simulink model "HybridModel_Phasor"  (R2018b)
settings: Solver=ode45  StartTime=0.0  StopTime=30  RelTol=1e-3
undefined symbols (not defined in the file or in its folder): A, B, C, D1, D11, Dd, Delta, j, to, V2G
libraries: powerlib x32, powerlib_meascontrol x28, simulink x2, re_lib x1
(part 1 of 4)
settings Model: Creator=Eduardo  LastModifiedBy=Eduardo

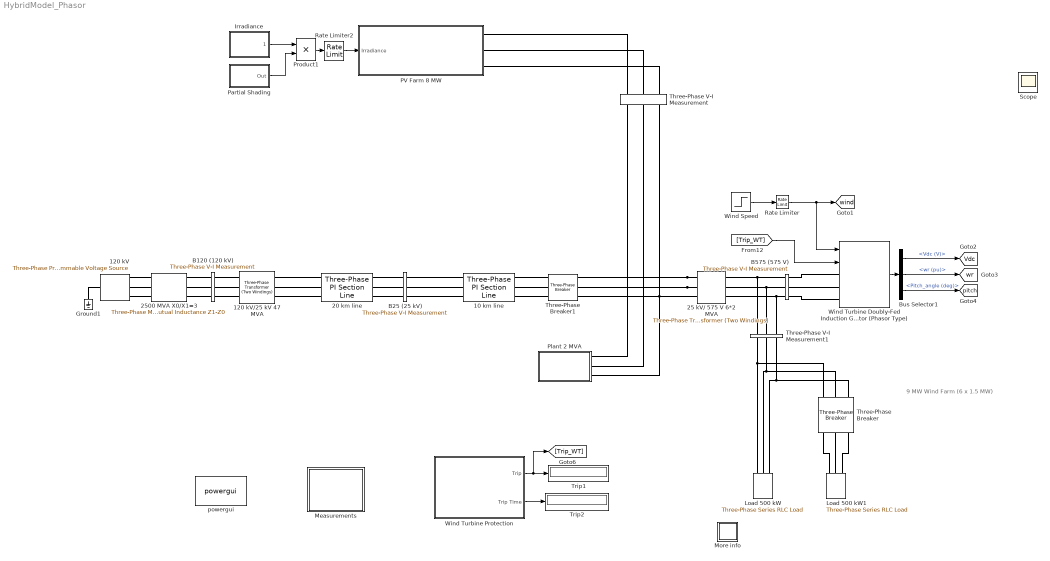
== system HybridModel_Phasor ==
  note: 9 MW Wind Farm
      | (6 x 1.5 MW)
  10 km line : powerlib/Elements/Three-Phase PI Section Line  LConnTagsString=a|b|c  RConnTagsString=A|B|C  Frequency=60  Resistances=[0.1153 0.413]  Inductances=[1.05e-3 3.32e-3]  Capacitances=[11.33e-009 5.01e-009]  Length=10
      settings: SourceProductName=Simscape Electrical
  120 kV : powerlib/Electrical Sources/Three-Phase Programmable Voltage Source  PositiveSequence=[120e3 0 60]  VariationEntity=None  VariationType=Step  VariationTypeAlt=Step  VariationStep=-0.15  VariationRate=10  VariationMagnitude=0.3  VariationFrequency=2  VariationTiming=[5 5.5]  VariationPhaseA=off  Amplitudes=[1 0.8 1.2 1.0]  TimeValues=[0 0.1 0.15 0.2]  HarmonicGeneration=off  HarmonicA=[1 -0.1 0 1]  HarmonicB=[2 0.15 35 2]  Timing="[5  5.5]"  BusType=swing  Pref=1e3  Qref=0  Qmin=-inf  Qmax=inf
      settings: SourceProductName=Simscape Electrical
  120 kV/25 kV 47 MVA : powerlib/Elements/Three-Phase Transformer (Two Windings)  Winding1Connection=Yg  Winding2Connection=Delta (D1)  CoreType=Three single-phase transformers  SetSaturation=off  Hysteresis=off  DataFile='basic_model'  SetInitialFlux=off  Measurements=None  UNITS=pu  NominalPower=[47e6 60 ]  Winding1="[ 120e3  0.08/30   0.08 ]"  Winding2="[ 25e3  0.08/30  0.08]"  Rm=500  Lm=500  L0=0.5  Saturation="[ 0,0  ;  0.005,1.2  ;  1.0,1.4 ]"  InitialFluxes=[ 0.8 , -0.8 , 0.7 ]  MoreParameters=off  BreakLoop=off  DataType=off  TransfoNumber=0
      settings: SourceProductName=Simscape Electrical
  20 km line : powerlib/Elements/Three-Phase PI Section Line  LConnTagsString=a|b|c  RConnTagsString=A|B|C  Frequency=60  Resistances=[0.1153 0.413]  Inductances=[1.05e-3 3.32e-3]  Capacitances=[11.33e-009 5.01e-009]  Length=20
      settings: SourceProductName=Simscape Electrical
  25 kV/ 575 V 6*2 MVA : powerlib/Elements/Three-Phase Transformer (Two Windings)  Winding1Connection=Yg  Winding2Connection=Delta (D1)  CoreType=Three single-phase transformers  SetSaturation=off  Hysteresis=off  DataFile='hysteresis'  SetInitialFlux=off  Measurements=None  UNITS=pu  NominalPower="[2e6*6  60]"  Winding1=[25e3 , 0.025/30 , 0.025]  Winding2=[ 575, 0.025/30 , 0.025]  Rm=500  Lm=inf  L0=0.5  Saturation=[ 0,0 ; 0.0024,1.2 ; 1.0,1.52 ]  InitialFluxes=[ 0.8 , -0.8 , 0.7 ]  MoreParameters=off  BreakLoop=off  DataType=off  TransfoNumber=0
      settings: SourceProductName=Simscape Electrical
  2500 MVA X0/X1=3 : powerlib/Elements/Three-Phase Mutual Inductance Z1-Z0  LConnTagsString=a|b|c  RConnTagsString=A|B|C  PositiveSequence="[0.1  1.0/(2*pi*60)] *120e3^2/2500e6"  ZeroSequence="[0.3  3.0/(2*pi*60)] *120e3^2/2500e6"
      settings: SourceProductName=Simscape Electrical  SourceProductBaseCode=PS
  B120 (120 kV) : powerlib/Measurements/Three-Phase V-I Measurement  VoltageMeasurement=phase-to-ground  SetLabelV=on  LabelV=Vabc_B120  Vpu=on  VpuLL=off  CurrentMeasurement=no  SetLabelI=on  LabelI=Iabc_B120  Ipu=off  Pbase=100e6  Vbase=120e3  OutputType=Complex  PhasorSimulation=on  PSBequivalent=0
      settings: SourceProductName=Simscape Electrical
  B25 (25 kV) : powerlib/Measurements/Three-Phase V-I Measurement  VoltageMeasurement=phase-to-ground  SetLabelV=on  LabelV=Vabc_B25  Vpu=on  VpuLL=off  CurrentMeasurement=yes  SetLabelI=on  LabelI=Iabc_B25  Ipu=on  Pbase=10e6  Vbase=25e3  OutputType=Complex  PhasorSimulation=on  PSBequivalent=0
      settings: SourceProductName=Simscape Electrical
  B575 (575 V) : powerlib/Measurements/Three-Phase V-I Measurement  VoltageMeasurement=phase-to-ground  SetLabelV=on  LabelV=Vabc_B575  Vpu=on  VpuLL=off  CurrentMeasurement=yes  SetLabelI=on  LabelI=Iabc_B575  Ipu=on  Pbase=6*1.5e6/0.9  Vbase=575  OutputType=Complex  PhasorSimulation=on  PSBequivalent=0
      settings: SourceProductName=Simscape Electrical
  Bus Selector1 : BusSelector  OutputSignals=Vdc (V),wr (pu),Pitch_angle (deg)
  Ground1 : powerlib/Elements/Ground  LConnTagsString=a
      settings: SourceProductName=Simscape Electrical
  Irradiance : Subsystem
      mask init:
      | load power_V2G
      mask Display: plot(V2G.IRRADIANCE.time,V2G.IRRADIANCE.SUN)
  Load 500 kW : powerlib/Elements/Three-Phase Series RLC Load  LConnTagsString=A|B|C  Configuration=Y (grounded)  NominalVoltage=575  Vabc=[1e3 1e3 1e3]  Vabcp=[1e3 1e3 1e3]  NominalFrequency=60  UnbalancedPower=off  ActivePower=500e3  InductivePower=0  CapacitivePower=0  Pabc=[10e3 9e3 11e3]  QLabc=[100 90 110]  QCabc=[100 90 110]  Pabcp=[10e3 9e3 11e3]  QLabcp=[100 90 110]  QCabcp=[100 90 110]  Measurements=None  LoadType=constant Z
      settings: SourceProductName=Simscape Electrical
  Load 500 kW1 : powerlib/Elements/Three-Phase Series RLC Load  LConnTagsString=A|B|C  Configuration=Y (grounded)  NominalVoltage=575  Vabc=[1e3 1e3 1e3]  Vabcp=[1e3 1e3 1e3]  NominalFrequency=60  UnbalancedPower=off  ActivePower=2e6  InductivePower=0  CapacitivePower=0  Pabc=[10e3 9e3 11e3]  QLabc=[100 90 110]  QCabc=[100 90 110]  Pabcp=[10e3 9e3 11e3]  QLabcp=[100 90 110]  QCabcp=[100 90 110]  Measurements=None  LoadType=constant Z
      settings: SourceProductName=Simscape Electrical
  Measurements : Subsystem
  More info : Subsystem
      settings: OpenFcn=showdemo(bdroot(gcb))
      mask Display: disp('?')
  PV Farm 8 MW : Subsystem  mask{eff=10, area=8e4}
      mask prompts: eff "Efficiency (%)"; area "Area (m^2)"
      mask help: The product of the effeciency, the area covered by the Pv farm and the irradiance in w/m2 will give you the power generate by the PV farm.
      mask DialogControl DescGroupVar Prompt: PV farm
      mask DialogControl DescTextVar Prompt: The product of the efficiency, the area covered by the PV farm and the irradiance in W/m2 will give you the power generated by the PV farm.
      mask Display: image(imread('panel.jpg'))
  Partial Shading : Subsystem  mask(Signal Disturbance){Hour=12, Minute=0, Second=0, Duration=5*60, Factor=0.7}
      mask prompts: Duration "Duration (s):"
      mask help: Within the specified time range defined by Start and Duration parameters, output is set to 'Factor'. Outside the specified time range output is kept at 1.0.
      mask init:
      | T2=(Hour-1)*60*60;    % Hour in seconds
      | T3=(Minute-1)*60;  % Minute in seconds
      | Ton=T2+T3+(Second-1);    % Beginning of fault (s)
      | Toff=Ton+Duration; % End of fault (s)
      mask TypeOptions Hour: 0 |      1 |      2 |      3 |      4 |      5 |      6 |      7 |      8 |      9 |     10 |     11 |     12 |     13 |     14 |     15 |     16 |     17 |     18 |     19 |     20 |     21 |     22 |     23
      mask TypeOptions Minute: 0 |      1 |      2 |      3 |      4 |      5 |      6 |      7 |      8 |      9 |     10 |     11 |     12 |     13 |     14 |     15 |     16 |     17 |     18 |     19 |     20 |     21 |     22 |     23 |     24 |     25 |     26 |     27 |     28 |     29 |     30 |     31 |     32 |     33 |     34 |     35 |     36 |     37 |     38 |     39 |     40 |     41 |     42 |     43 |     44 |     45 |     46 |     47 |     48 |     49 |     50 |     51 |     52 |     53 |     54 |     55 |     56 |     57 |     58 |     59
      mask TypeOptions Second: 0 |      1 |      2 |      3 |      4 |      5 |      6 |      7 |      8 |      9 |     10 |     11 |     12 |     13 |     14 |     15 |     16 |     17 |     18 |     19 |     20 |     21 |     22 |     23 |     24 |     25 |     26 |     27 |     28 |     29 |     30 |     31 |     32 |     33 |     34 |     35 |     36 |     37 |     38 |     39 |     40 |     41 |     42 |     43 |     44 |     45 |     46 |     47 |     48 |     49 |     50 |     51 |     52 |     53 |     54 |     55 |     56 |     57 |     58 |     59
      mask DialogControl Control2 Prompt: Start:
  Plant 2 MVA : Subsystem
  Product1 : Product
  Rate Limiter : RateLimiter
  Rate Limiter2 : RateLimiter  RisingSlewLimit=1e4  FallingSlewLimit=-1e4  SampleTimeMode=inherited
  Scope : Scope  NumInputPorts=3
  Three-Phase V-I Measurement : powerlib/Measurements/Three-Phase V-I Measurement  VoltageMeasurement=phase-to-ground  SetLabelV=on  LabelV=V_PV  Vpu=off  VpuLL=off  CurrentMeasurement=yes  SetLabelI=on  LabelI=I_PV  Ipu=off  Pbase=100e6  Vbase=500e3  OutputType=Complex  PhasorSimulation=on  PSBequivalent=0
  Three-Phase V-I Measurement1 : powerlib/Measurements/Three-Phase V-I Measurement  VoltageMeasurement=phase-to-ground  SetLabelV=on  LabelV=Vabc_load  Vpu=off  VpuLL=off  CurrentMeasurement=yes  SetLabelI=on  LabelI=Iabc_load  Ipu=off  Pbase=100e6  Vbase=500e3  OutputType=Complex  PhasorSimulation=on  PSBequivalent=0
  Three-Phase Breaker : powerlib/Elements/Three-Phase Breaker  InitialState=open  SwitchA=on  SwitchB=on  SwitchC=on  SwitchTimes=[5 15]  External=off  BreakerResistance=0.01  SnubberResistance=1e6  SnubberCapacitance=inf  Measurements=None
  Three-Phase Breaker1 : powerlib/Elements/Three-Phase Breaker  InitialState=closed  SwitchA=on  SwitchB=on  SwitchC=on  SwitchTimes="[20  60]"  External=off  BreakerResistance=0.01  SnubberResistance=1e6  SnubberCapacitance=inf  Measurements=None
  Trip1 : Display
  Trip2 : Display
  Wind Speed : Step  Time=5  Before=8  After=8  SampleTime=0
  Wind Turbine Doubly-Fed Induction Generator (Phasor Type) : re_lib/Wind Generation/Wind Turbine Doubly-Fed Induction Generator (Phasor Type)  ExternalTm=off  nom=[6*1.5e6/0.9 575 60]  sta=[ 0.00706 0.171]  rot=[ 0.005 0.156]  Lm=2.9  mec=[5.04 0.01 3]  init=[0.2 0 0 0 0 0]  speed_power=[0 0; 0.24 0.007; 0.36 0.024; 0.6 0.112; 0.96 0.46; 1.2 0.898; 1.5 0.898]  Pmec=6*1.5e6  speed_ABCD=[0.7 0.71 1.2 1.21]  power_C=0.73  wind_point_C=12  pitch_gain=500  pitch_max=45  pitch_rate=2  Pmax=0.5  Lchoke=[0.15 0.15/100]  init_inductor=[0 90]  Vdc_nom=1200  capacitor=6*10000e-6  ControlVQ=Voltage regulation  Vref=1.0  ExternalVref=off  Qref=0  ExternalQref=off  Iq_ref=0  ExternalIqref=off  Kpi_volt_reg=[1.25 300]  Xs=0.02  Kpi_Q=[0.05 5]  Kpi_power_reg=[1 100]  Kpi_dc_reg=[0.002 0.05]  Kpi_grid_side_cur_reg=[1 100]  Kpi_rotor_side_cur_reg=[0.3 8]  V_slew_rate=100  Q_slew_rate=100  power_slew_rate=1  current_slew_rate=200
      settings: SourceProductName=Simscape Electrical  SourceProductBaseCode=PS
  Wind Turbine Protection : Subsystem
      mask Display: disp('Wind\nTurbine\nProtection')
  powergui : powerlib/powergui  Priority=2  SimulationMode=Phasor  SampleTime=5e-6  frequency=60  Iterations=50  frequencyindice=60  Pbase=100e6  ErrMax=1e-4  UnitsV=kV  UnitsW=MW  buscounter=0  FunctionMessages=off  echomessages=off  EnableUseOfTLC=off  CurrentSourceSwitches=off  DisableSnubberDevices=off  DisableRonSwitches=off  DisableVfSwitches=off  DisplayEquations=off  SolverType=Tustin/Backward Euler (TBE)  Interpol=off  ExternalGateDelay=off  methode=off  Ts=100  x0status=blocks  SPID=off  SwTol=0  HookPort=off  RestoreLinks=warning  ResistiveCurrentMeasurement=off  Frange=[0:2:500]  Ylog=off  Xlog=off  ShowGrid=off  save=off  variable=ZData  structure=0  ZoomFFT=on  StartTime=0.0  cycles=1  DisplayStyle=1  fundamental=60  FreqAxis=off  MaxFrequency=1000  frequencyindicesteady=1  RmsSteady=1  display=off
  tag scope: Vdc=global, pitch=global, wind=global, wr=global
  wires:
  Wind Speed/1 -> Rate Limiter/1
  Rate Limiter/1 -> Wind Turbine Doubly-Fed Induction Generator (Phasor Type)/1, [wind]
  Wind Turbine Protection/2(Trip Time) -> Trip2/1
  Wind Turbine Protection/1(Trip) -> [Trip_WT], Trip1/1
  Wind Turbine Doubly-Fed Induction Generator (Phasor Type)/1 -> Bus Selector1/1
  Bus Selector1/2 -> [wr]  "<wr (pu)>"
  Bus Selector1/1 -> [Vdc]  "<Vdc (V)>"
  Bus Selector1/3 -> [pitch]  "<Pitch_angle (deg)>"
  [Trip_WT] -> Wind Turbine Doubly-Fed Induction Generator (Phasor Type)/2
  ? -> ?
  Product1/1 -> Rate Limiter2/1
  Rate Limiter2/1 -> PV Farm 8 MW/1(Irradiance)
  Partial Shading/1(Out) -> Product1/2
  Irradiance/1(" ") -> Product1/1
  connections:
  B25 (25 kV)/RConn1 -- 10 km line/LConn1
  B25 (25 kV)/RConn2 -- 10 km line/LConn2
  B25 (25 kV)/RConn3 -- 10 km line/LConn3
  B575 (575 V)/LConn2 -- Three-Phase V-I Measurement1/RConn2 -- 25 kV/ 575 V 6*2 MVA/RConn2
  B575 (575 V)/LConn1 -- Three-Phase V-I Measurement1/RConn1 -- 25 kV/ 575 V 6*2 MVA/RConn1
  120 kV/25 kV 47 MVA/RConn2 -- 20 km line/LConn2
  120 kV/25 kV 47 MVA/RConn3 -- 20 km line/LConn3
  Load 500 kW/LConn3 -- Three-Phase V-I Measurement1/LConn3 -- Three-Phase Breaker/RConn3
  120 kV/25 kV 47 MVA/RConn1 -- 20 km line/LConn1
  B25 (25 kV)/LConn1 -- 20 km line/RConn1
  B575 (575 V)/RConn2 -- Wind Turbine Doubly-Fed Induction Generator (Phasor Type)/LConn2
  120 kV/RConn1 -- 2500 MVA X0/X1=3/LConn1
  B120 (120 kV)/RConn2 -- 120 kV/25 kV 47 MVA/LConn2
  B120 (120 kV)/LConn2 -- 2500 MVA X0/X1=3/RConn2
  B120 (120 kV)/LConn3 -- 2500 MVA X0/X1=3/RConn3
  B120 (120 kV)/RConn1 -- 120 kV/25 kV 47 MVA/LConn1
  20 km line/RConn3 -- B25 (25 kV)/LConn3
  B575 (575 V)/RConn1 -- Wind Turbine Doubly-Fed Induction Generator (Phasor Type)/LConn1
  120 kV/RConn3 -- 2500 MVA X0/X1=3/LConn3
  B575 (575 V)/RConn3 -- Wind Turbine Doubly-Fed Induction Generator (Phasor Type)/LConn3
  120 kV/RConn2 -- 2500 MVA X0/X1=3/LConn2
  20 km line/RConn2 -- B25 (25 kV)/LConn2
  Ground1/LConn1 -- 120 kV/LConn1
  B120 (120 kV)/LConn1 -- 2500 MVA X0/X1=3/RConn1
  B120 (120 kV)/RConn3 -- 120 kV/25 kV 47 MVA/LConn3
  Plant 2 MVA/LConn3 -- 25 kV/ 575 V 6*2 MVA/LConn3 -- Three-Phase Breaker1/RConn3 -- Three-Phase V-I Measurement/RConn3
  25 kV/ 575 V 6*2 MVA/LConn1 -- Plant 2 MVA/LConn1 -- Three-Phase Breaker1/RConn1 -- Three-Phase V-I Measurement/RConn1
  25 kV/ 575 V 6*2 MVA/LConn2 -- Plant 2 MVA/LConn2 -- Three-Phase Breaker1/RConn2 -- Three-Phase V-I Measurement/RConn2
  Load 500 kW1/LConn1 -- Three-Phase Breaker/LConn1
  Load 500 kW1/LConn2 -- Three-Phase Breaker/LConn2
  Load 500 kW1/LConn3 -- Three-Phase Breaker/LConn3
  PV Farm 8 MW/RConn1 -- Three-Phase V-I Measurement/LConn1
  PV Farm 8 MW/RConn2 -- Three-Phase V-I Measurement/LConn2
  PV Farm 8 MW/RConn3 -- Three-Phase V-I Measurement/LConn3
  Three-Phase Breaker1/LConn1 -- 10 km line/RConn1
  Three-Phase Breaker1/LConn3 -- 10 km line/RConn3
  Three-Phase Breaker1/LConn2 -- 10 km line/RConn2
  Load 500 kW/LConn1 -- Three-Phase V-I Measurement1/LConn1 -- Three-Phase Breaker/RConn1
  Load 500 kW/LConn2 -- Three-Phase V-I Measurement1/LConn2 -- Three-Phase Breaker/RConn2
  B575 (575 V)/LConn3 -- Three-Phase V-I Measurement1/RConn3 -- 25 kV/ 575 V 6*2 MVA/RConn3

== system HybridModel_Phasor/Irradiance ==
  1-D Lookup IRRADIANCE Table : Lookup_n-D  NumberOfTableDimensions=1  BreakpointsForDimension1=V2G.IRRADIANCE.time  BeginIndexSearchUsingPreviousIndexResult=on  Table=V2G.IRRADIANCE.SUN  InternalRulePriority=Speed  RndMeth=Simplest  InputSameDT=on
  Add : Sum
  Clock1 : Clock
  Constant1 : Constant
  Second-->Hour : Gain  Gain=1/(60*60)
  " " : Outport
  wires:
  Constant1/1 -> Add/2
  Add/1 -> 1-D Lookup IRRADIANCE Table/1  "Hour of the day"
  1-D Lookup IRRADIANCE Table/1 -> " "/1
  Clock1/1 -> Second-->Hour/1
  Second-->Hour/1 -> Add/1

== system HybridModel_Phasor/Measurements ==
  Grid : Scope  NumInputPorts=8
  Grid Data acquisition : Subsystem
  PV : Scope  NumInputPorts=4
  PV Array DATA : Subsystem
  Wind Turbine : Scope  NumInputPorts=8
  Wind turbine Data acquisition : Subsystem
  wires:
  Wind turbine Data acquisition/3(P_mean) -> Wind Turbine/3  "Generated P(MW)"
  Grid Data acquisition/1("Vabc_B120 ") -> Grid/1  "Vabc_B120 (pu)"
  Grid Data acquisition/2("Vabc_B25 ") -> Grid/2  "Vabc_B25 (pu)"
  Grid Data acquisition/3("Vabc_B575 ") -> Grid/3  "Vabc_B575 (pu)"
  Grid Data acquisition/4(P_B25) -> Grid/4  "P_B25 (MW)"
  Grid Data acquisition/5(Q_B25) -> Grid/5  "Q_B25 (Mvar)"
  [Vdc] -> Wind Turbine/5  "Vdc (V)"
  [wr] -> Wind Turbine/6  "Speed (pu)"
  Wind turbine Data acquisition/1(V1_B575) -> Wind Turbine/1  "Pos. seq. V1_B575 (pu)"
  Wind turbine Data acquisition/2(I1_B575) -> Wind Turbine/2  "Pos. seq. I1_B575 (pu)"
  Wind turbine Data acquisition/4(Q_mean) -> Wind Turbine/4  "Generated Q(Mvar)"
  Grid Data acquisition/8(Motor_Speed) -> Grid/8  "Motor Speed (pu)"
  Grid Data acquisition/7(I1_Plant) -> Grid/7  "I Plant pos. seq. (pu/2 MVA)"
  Grid Data acquisition/6(V1_Plant) -> Grid/6  "V_Plant 2.3kV pos. seq. (pu)"
  [wind] -> Wind Turbine/7  "Wind speed (m/s)"
  [pitch] -> Wind Turbine/8  "pitch angle (deg)"
  PV Array DATA/2(I_PV) -> PV/2  "Pos. seq. I1_B575 (pu)"
  PV Array DATA/3(P_mean) -> PV/3  "Generated P(MW)"
  PV Array DATA/4(Q_mean) -> PV/4  "Generated Q(Mvar)"
  PV Array DATA/1(V_PV) -> PV/1  "Pos. seq. V1_B575 (pu)"

== system HybridModel_Phasor/More info ==

== system HybridModel_Phasor/PV Farm 8 MW ==
  Irradiance : Inport
  PV Farm : Subsystem
  PV farm : Scope  NumInputPorts=2
  "Power (3ph, Phasor)2" : powerlib_meascontrol/Measurements/Power (3ph, Phasor)
      settings: SourceProductName=Simscape Power Systems  SourceProductBaseCode=PS
  VabcPV : powerlib/Measurements/Three-Phase V-I Measurement  VoltageMeasurement=phase-to-ground  SetLabelV=on  LabelV=V_Solar  Vpu=off  VpuLL=off  CurrentMeasurement=yes  SetLabelI=on  LabelI=I_Solar  Ipu=off  Pbase=2*1.5e6/0.9  Vbase=25e3  OutputType=Complex  PhasorSimulation=on  PSBequivalent=0
  A : PMIOPort  Side=Right
  B : PMIOPort  Port=2  Side=Right
  C : PMIOPort  Port=3  Side=Right
  tag scope: Solar_Power=global
  wires:
  Irradiance/1 -> PV Farm/1(irradiance)
  [V_Solar] -> "Power (3ph, Phasor)2"/1
  "Power (3ph, Phasor)2"/1 -> [Solar_Power], PV farm/1  "P(W)"
  [I_Solar] -> "Power (3ph, Phasor)2"/2
  "Power (3ph, Phasor)2"/2 -> PV farm/2  "Q(VA)"
  connections:
  B/RConn1 -- VabcPV/RConn2
  VabcPV/LConn2 -- PV Farm/RConn2
  A/RConn1 -- VabcPV/RConn1
  VabcPV/RConn3 -- C/RConn1
  PV Farm/RConn1 -- VabcPV/LConn1
  VabcPV/LConn3 -- PV Farm/RConn3

== system HybridModel_Phasor/Partial Shading ==
  Add : Sum
  Clock : Clock
  Compare To Constant : simulink/Logic and Bit Operations/Compare To Constant  relop=>=  const=Ton  OutDataTypeStr=boolean
  Compare To Constant1 : simulink/Logic and Bit Operations/Compare To Constant  relop=<  const=Toff  OutDataTypeStr=boolean
  Constant : Constant  Value=Factor
  Logical Operator : Logic  AllPortsSameDT=off  OutDataTypeStr=float('double')
  Logical Operator1 : Logic  Operator=NOT  AllPortsSameDT=off  OutDataTypeStr=float('double')
  Product : Product
  Out : Outport
  wires:
  Add/1 -> Out/1
  Product/1 -> Add/2
  Constant/1 -> Product/2
  Compare To Constant/1 -> Logical Operator/1
  Clock/1 -> Compare To Constant1/1, Compare To Constant/1
  Compare To Constant1/1 -> Logical Operator/2
  Logical Operator/1 -> Logical Operator1/1, Product/1
  Logical Operator1/1 -> Add/1

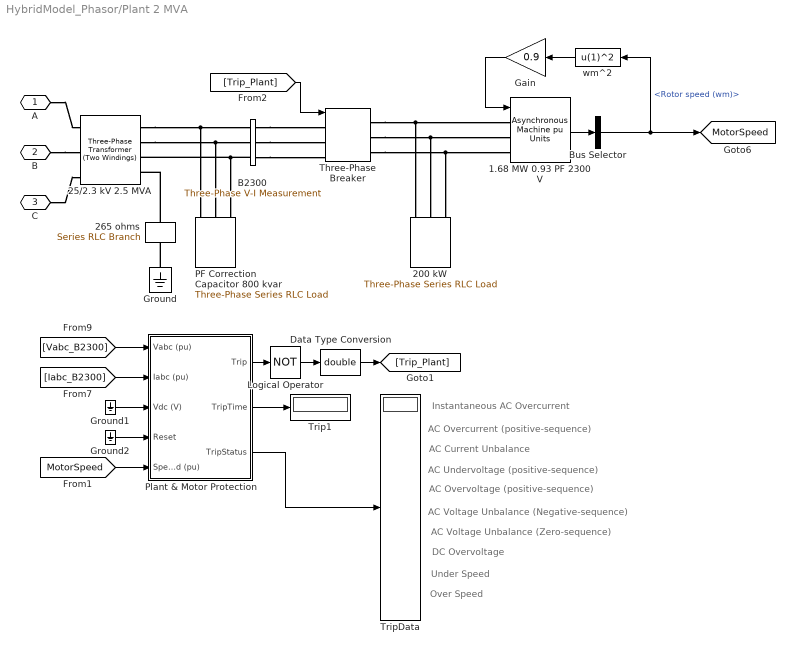
== system HybridModel_Phasor/Plant 2 MVA ==
  note: Instantaneous AC Overcurrent
  note: AC Overcurrent (positive-sequence)
  note: AC Current Unbalance
  note: AC Undervoltage (positive-sequence)
  note: AC Overvoltage (positive-sequence)
  note: AC Voltage Unbalance (Negative-sequence)
  note: AC Voltage Unbalance (Zero-sequence)
  note: DC Overvoltage
  note: Under Speed
  note: Over Speed
  1.68 MW 0.93 PF 2300 V : powerlib/Machines/Asynchronous Machine pu Units  RotorType=Squirrel-cage  PresetModel=No  MechanicalLoad=Torque Tm  ShowDetailedParameters=on  ReferenceFrame=Rotor  Units=pu  MeasurementBus=off  NominalParameters=[1.68e6/0.93 2300 60]  Stator=[0.0092 0.0717]  Rotor=[0.007 0.0717]  Cage1=[0.01909 0.0397]  Cage2=[0.01909 0.0397]  Lm=4.14  Mechanical=[0.5 0 2]  PolePairs=2  InitialConditions="[ 1e-3,0   0,0,0   0,0,0 ]"  SimulateSaturation=off  Saturation=[ 0 0 ; 0 0 ]  LoadFlowParameters=0  TsPowergui=0  TsBlock=-1  IterativeModel=Forward Euler  IterativeDiscreteModel=Trapezoidal non iterative  Pmec=3e3
      settings: SourceProductName=Simscape Electrical  SourceProductBaseCode=PS
  200 kW : powerlib/Elements/Three-Phase Series RLC Load  LConnTagsString=A|B|C  Configuration=Y (grounded)  NominalVoltage=2300  Vabc=[1e3 1e3 1e3]  Vabcp=[1e3 1e3 1e3]  NominalFrequency=60  UnbalancedPower=off  ActivePower=200e3  InductivePower=0  CapacitivePower=0  Pabc=[10e3 9e3 11e3]  QLabc=[100 90 110]  QCabc=[100 90 110]  Pabcp=[10e3 9e3 11e3]  QLabcp=[100 90 110]  QCabcp=[100 90 110]  Measurements=None  LoadType=constant Z
      settings: SourceProductName=Simscape Electrical
  25/2.3 kV 2.5 MVA : powerlib/Elements/Three-Phase Transformer (Two Windings)  Winding1Connection=Delta (D11)  Winding2Connection=Yn  CoreType=Three single-phase transformers  SetSaturation=off  Hysteresis=off  DataFile='basic_model'  SetInitialFlux=off  Measurements=None  UNITS=pu  NominalPower=[2.5e6 60 ]  Winding1="[ 25e3  0.04/30   0.04 ]"  Winding2="[ 2.3e3  0.04/30  0.04]"  Rm=500  Lm=500  L0=0.5  Saturation="[ 0,0  ;  0.005,1.2  ;  1.0,1.4 ]"  InitialFluxes=[ 0.8 , -0.8 , 0.7 ]  MoreParameters=off  BreakLoop=off  DataType=off  TransfoNumber=0
      settings: SourceProductName=Simscape Electrical
  265 ohms : powerlib/Elements/Series RLC Branch  LConnTagsString=__new0  RConnTagsString=__new0  BranchType=R  Resistance=265  Inductance=1.0  SetiL0=off  InitialCurrent=0  Capacitance=1.0  Setx0=off  InitialVoltage=0  Measurements=None
      settings: SourceProductName=Simscape Electrical
  B2300 : powerlib/Measurements/Three-Phase V-I Measurement  VoltageMeasurement=phase-to-ground  SetLabelV=on  LabelV=Vabc_B2300  Vpu=on  VpuLL=off  CurrentMeasurement=yes  SetLabelI=on  LabelI=Iabc_B2300  Ipu=on  Pbase=2.0e6  Vbase=2300  OutputType=Complex  PhasorSimulation=on  PSBequivalent=0
      settings: SourceProductName=Simscape Electrical
  Bus Selector : BusSelector  OutputSignals=Mechanical.Rotor speed (wm)
  Data Type Conversion : DataTypeConversion  OutDataTypeStr=double  SampleTime=0  SaturateOnIntegerOverflow=on  RndMeth=Zero
  Gain : Gain  Gain=0.9  SaturateOnIntegerOverflow=on  OutDataTypeStr=Inherit: Same as input  ParamDataTypeStr=Inherit: Same as input
  Ground : powerlib/Elements/Ground  LConnTagsString=a
      settings: SourceProductName=Simscape Electrical
  Ground1 : Ground
  Ground2 : Ground
  Logical Operator : Logic  Operator=NOT  AllPortsSameDT=off
  PF Correction Capacitor 800 kvar : powerlib/Elements/Three-Phase Series RLC Load  LConnTagsString=A|B|C  Configuration=Y (grounded)  NominalVoltage=2300  Vabc=[1e3 1e3 1e3]  Vabcp=[1e3 1e3 1e3]  NominalFrequency=60  UnbalancedPower=off  ActivePower=0  InductivePower=0  CapacitivePower=800e3  Pabc=[10e3 9e3 11e3]  QLabc=[100 90 110]  QCabc=[100 90 110]  Pabcp=[10e3 9e3 11e3]  QLabcp=[100 90 110]  QCabcp=[100 90 110]  Measurements=None  LoadType=constant Z
      settings: SourceProductName=Simscape Electrical
  Plant & Motor Protection : Subsystem  mask(Protection System){Freq=60, Max_Iinst=10, MaxI1=[ 1.1, 5 ], MaxI2I1=[ 0.4, 0.2], MinMaxV1=[ 0.9, 1.1, 0.2 ], MaxV2V1=[ 0.1, 0.1, 0.3 ], MaxVdc=[ inf, 0 ], MaxSpeed=[ 0.9, 1.1, 1 ], Delay_Protection=1}
      mask prompts: Freq "Fundamental frequency f1 (Hz):"; Max_Iinst "Instantaneous AC Overcurrent (pu):"; MaxI1 "Maximum AC Current [ I1max(pu), Delay(s) ]:"; MaxI2I1 "Maximum AC Current Unbalance [ I2/I1max(pu), Delay(s) ]"; MinMaxV1 "AC Under/Over Voltage [ V1min(pu), V1max(pu), Delay(s) ]:"; MaxV2V1 "Maximum Voltage Unbalance [ V2/V1max(pu), V0/V1max(pu), Delay(s)]:"; MaxVdc "Maximum DC Voltage  [ Vmax(V), Delay(s) ]:"; MaxSpeed "Under/Over Speed [ Speedmin (pu), Speedmax (pu), Delay(s)]:"; Delay_Protection "Start time for protection system (s):"
      mask help:
      | Protection type:
      | 1.    Instantaneous AC Overcurrent
      | 2.    AC Overcurrent (positive-sequence)
      | 3.    AC Current Unbalance
      | 4.    AC Undervoltage (positive-sequence)
      | 5.    AC Overvoltage (positive-sequence)
      | 6.    AC Voltage Unbalance (Negative-sequence)
      | 7.    AC Voltage Unbalance (Zero-sequence)
      | 8.    DC Overvoltage
      | 9.    Under Speed
      | 10.  Over Speed
      mask init:
      | a=exp(2*pi*j/3);
      | a2=a^2;
      | Max_I1=MaxI1(1);
      | Delay_I1=MaxI1(2);
      | Max_I2_I1=MaxI2I1(1);
      | Delay_I2_I1=MaxI2I1(2);
      | Min_V1=MinMaxV1(1);
      | Max_V1=MinMaxV1(2);
      | Delay_V1=MinMaxV1(3);
      | Max_V2_V1=MaxV2V1(1);
      | Max_V0_V1=MaxV2V1(2);
      | Delay_V2_V1=MaxV2V1(3);
      | Max_Vdc=MaxVdc(1);
      | Delay_Vdc=MaxVdc(2);
      | Min_Speed=MaxSpeed(1);
      | Max_Speed=MaxSpeed(2);
      | Delay_Speed=MaxSpeed(3);
  Three-Phase Breaker : powerlib/Elements/Three-Phase Breaker  InitialState=closed  SwitchA=on  SwitchB=on  SwitchC=on  SwitchTimes="[4/60  10/60]"  External=on  BreakerResistance=0.001  SnubberResistance=inf  SnubberCapacitance=inf  Measurements=None
      settings: SourceProductName=Simscape Electrical
  Trip1 : Display
  TripData : Display
  wm^2 : Fcn  Expr=u(1)^2
  A : PMIOPort  Side=Left
  B : PMIOPort  Port=2  Side=Left
  C : PMIOPort  Port=3  Side=Left
  tag scope: MotorSpeed=global
  wires:
  1.68 MW 0.93 PF 2300 V/1 -> Bus Selector/1
  Bus Selector/1 -> wm^2/1, [MotorSpeed]  "<Rotor speed (wm)>"
  wm^2/1 -> Gain/1
  [Vabc_B2300] -> Plant & Motor Protection/1(Vabc (pu))
  [Iabc_B2300] -> Plant & Motor Protection/2(Iabc (pu))
  Ground1/1 -> Plant & Motor Protection/3(Vdc (V))
  Ground2/1 -> Plant & Motor Protection/4(Reset)
  [MotorSpeed] -> Plant & Motor Protection/5(Speed (pu))
  Plant & Motor Protection/1(Trip) -> Logical Operator/1
  [Trip_Plant] -> Three-Phase Breaker/1
  Plant & Motor Protection/2(TripTime) -> Trip1/1
  Plant & Motor Protection/3(TripStatus) -> TripData/1
  Data Type Conversion/1 -> [Trip_Plant]
  Logical Operator/1 -> Data Type Conversion/1
  Gain/1 -> 1.68 MW 0.93 PF 2300 V/1
  connections:
  265 ohms/LConn1 -- 25/2.3 kV 2.5 MVA/RConn4
  Ground/LConn1 -- 265 ohms/RConn1
  A/RConn1 -- 25/2.3 kV 2.5 MVA/LConn1
  B/RConn1 -- 25/2.3 kV 2.5 MVA/LConn2
  C/RConn1 -- 25/2.3 kV 2.5 MVA/LConn3
  25/2.3 kV 2.5 MVA/RConn1 -- B2300/LConn1 -- PF Correction Capacitor 800 kvar/LConn1
  25/2.3 kV 2.5 MVA/RConn2 -- B2300/LConn2 -- PF Correction Capacitor 800 kvar/LConn2
  B2300/LConn3 -- 25/2.3 kV 2.5 MVA/RConn3 -- PF Correction Capacitor 800 kvar/LConn3
  B2300/RConn1 -- Three-Phase Breaker/LConn1
  B2300/RConn2 -- Three-Phase Breaker/LConn2
  B2300/RConn3 -- Three-Phase Breaker/LConn3
  Three-Phase Breaker/RConn1 -- 1.68 MW 0.93 PF 2300 V/LConn1 -- 200 kW/LConn1
  Three-Phase Breaker/RConn2 -- 1.68 MW 0.93 PF 2300 V/LConn2 -- 200 kW/LConn2
  Three-Phase Breaker/RConn3 -- 1.68 MW 0.93 PF 2300 V/LConn3 -- 200 kW/LConn3

== system HybridModel_Phasor/Wind Turbine Protection ==
  note: Instantaneous AC Overcurrent
  note: AC Overcurrent (positive-sequence)
  note: AC Current Unbalance
  note: AC Undervoltage (positive-sequence)
  note: AC Overvoltage (positive-sequence)
  note: AC Voltage Unbalance (Negative-sequence)
  note: AC Voltage Unbalance (Zero-sequence)
  note: DC Overvoltage
  note: Under Speed
  note: Over Speed
  Ground2 : Ground
  Protection System : Subsystem  mask(Protection System){Freq=60, Max_Iinst=10, MaxI1=[ 1.1, 5 ], MaxI2I1=[ 0.4, 0.2], MinMaxV1=[ 0.75, 1.1, 0.1 ], MaxV2V1=[ 0.05, 0.05, 0.2 ], MaxVdc=[ 1900, 0.001 ], MaxSpeed=[ 0.3, 1.5, 5 ], Delay_Protection=5}
      mask prompts: Freq "Fundamental frequency f1 (Hz):"; Max_Iinst "Instantaneous AC Overcurrent (pu):"; MaxI1 "Maximum AC Current [ I1max(pu), Delay(s) ]:"; MaxI2I1 "Maximum AC Current Unbalance [ I2/I1max(pu), Delay(s) ]"; MinMaxV1 "AC Under/Over Voltage [ V1min(pu), V1max(pu), Delay(s) ]:"; MaxV2V1 "Maximum Voltage Unbalance [ V2/V1max(pu), V0/V1max(pu), Delay(s)]:"; MaxVdc "Maximum DC Voltage  [ Vmax(V), Delay(s) ]:"; MaxSpeed "Under/Over Speed [ Speedmin (pu), Speedmax (pu), Delay(s)]:"; Delay_Protection "Start time for protection system (s):"
      mask help:
      | Protection type:
      | 1.    Instantaneous AC Overcurrent
      | 2.    AC Overcurrent (positive-sequence)
      | 3.    AC Current Unbalance
      | 4.    AC Undervoltage (positive-sequence)
      | 5.    AC Overvoltage (positive-sequence)
      | 6.    AC Voltage Unbalance (Negative-sequence)
      | 7.    AC Voltage Unbalance (Zero-sequence)
      | 8.    DC Overvoltage
      | 9.    Under Speed
      | 10.  Over Speed
      mask init: same as HybridModel_Phasor/Plant 2 MVA/Plant & Motor Protection
  TripData : Display
  Trip : Outport
  Trip Time : Outport  Port=2
  wires:
  Ground2/1 -> Protection System/4(Reset)
  Protection System/3(TripStatus) -> TripData/1
  [Vabc_B575] -> Protection System/1(Vabc (pu))
  [Vdc] -> Protection System/3(Vdc (V))
  [wr] -> Protection System/5(Speed (pu))
  [Iabc_B575] -> Protection System/2(Iabc (pu))
  Protection System/1(Trip) -> Trip/1
  Protection System/2(TripTime) -> Trip Time/1

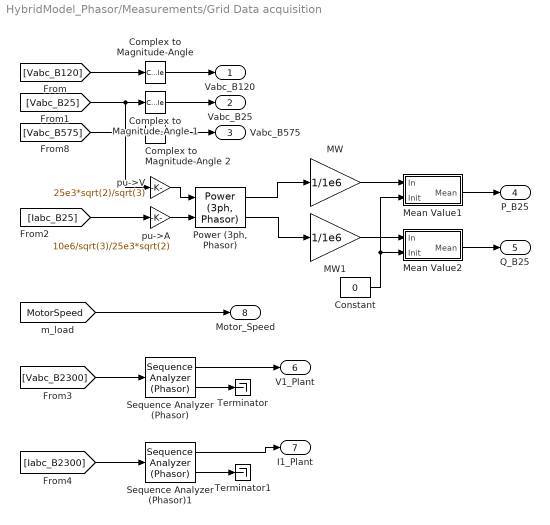
== system HybridModel_Phasor/Measurements/Grid Data acquisition ==
  "Complex to Magnitude-Angle " : ComplexToMagnitudeAngle  Output=Magnitude
  Complex to Magnitude-Angle 1 : ComplexToMagnitudeAngle  Output=Magnitude
  Complex to Magnitude-Angle 2 : ComplexToMagnitudeAngle  Output=Magnitude
  Constant : Constant  Value=0
  MW : Gain  Gain=1/1e6  SaturateOnIntegerOverflow=on  OutDataTypeStr=Inherit: Same as input  ParamDataTypeStr=Inherit: Same as input
  MW1 : Gain  Gain=1/1e6  SaturateOnIntegerOverflow=on  OutDataTypeStr=Inherit: Same as input  ParamDataTypeStr=Inherit: Same as input
  Mean Value1 : Subsystem  mask(Mean value){Period=1/60}
      mask prompts: Period "Averaging period (s):"
      mask help: This block uses the running window averaging technique to compute the mean value of the input signal over the specified period.
  Mean Value2 : Subsystem  mask(Mean value){Period=1/60}
      mask prompts: Period "Averaging period (s):"
      mask help: This block uses the running window averaging technique to compute the mean value of the input signal over the specified period.
  "Power (3ph, Phasor)" : powerlib_meascontrol/Measurements/Power (3ph, Phasor)
      settings: SourceProductName=Simscape Electrical  SourceProductBaseCode=PS
  Sequence Analyzer (Phasor) : powerlib_meascontrol/Measurements/Sequence Analyzer (Phasor)  seq=Positive
      settings: SourceProductName=Simscape Electrical  SourceProductBaseCode=PS
  Sequence Analyzer (Phasor)1 : powerlib_meascontrol/Measurements/Sequence Analyzer (Phasor)  seq=Positive
      settings: SourceProductName=Simscape Electrical  SourceProductBaseCode=PS
  Terminator : Terminator
  Terminator1 : Terminator
  pu->A : Gain  Gain=10e6/sqrt(3)/25e3*sqrt(2)  SaturateOnIntegerOverflow=on  OutDataTypeStr=Inherit: Same as input  ParamDataTypeStr=Inherit: Same as input
  pu->V : Gain  Gain=25e3*sqrt(2)/sqrt(3)  SaturateOnIntegerOverflow=on  OutDataTypeStr=Inherit: Same as input  ParamDataTypeStr=Inherit: Same as input
  "Vabc_B120 " : Outport
  "Vabc_B25 " : Outport  Port=2
  "Vabc_B575 " : Outport  Port=3
  P_B25 : Outport  Port=4
  Q_B25 : Outport  Port=5
  V1_Plant : Outport  Port=6
  I1_Plant : Outport  Port=7
  Motor_Speed : Outport  Port=8
  wires:
  pu->A/1 -> "Power (3ph, Phasor)"/2
  pu->V/1 -> "Power (3ph, Phasor)"/1
  "Complex to Magnitude-Angle "/1 -> "Vabc_B120 "/1
  [Vabc_B120] -> "Complex to Magnitude-Angle "/1
  Complex to Magnitude-Angle 1/1 -> "Vabc_B25 "/1
  [Vabc_B25] -> Complex to Magnitude-Angle 1/1, pu->V/1
  Complex to Magnitude-Angle 2/1 -> "Vabc_B575 "/1
  [Vabc_B575] -> Complex to Magnitude-Angle 2/1
  [Iabc_B25] -> pu->A/1
  Constant/1 -> Mean Value1/2(Init), Mean Value2/2(Init)
  Mean Value1/1(Mean) -> P_B25/1
  Mean Value2/1(Mean) -> Q_B25/1
  [MotorSpeed] -> Motor_Speed/1
  [Vabc_B2300] -> Sequence Analyzer (Phasor)/1
  Sequence Analyzer (Phasor)/1 -> V1_Plant/1
  Sequence Analyzer (Phasor)/2 -> Terminator/1
  [Iabc_B2300] -> Sequence Analyzer (Phasor)1/1
  Sequence Analyzer (Phasor)1/1 -> I1_Plant/1
  Sequence Analyzer (Phasor)1/2 -> Terminator1/1
  MW/1 -> Mean Value1/1(In)
  MW1/1 -> Mean Value2/1(In)
  "Power (3ph, Phasor)"/1 -> MW/1
  "Power (3ph, Phasor)"/2 -> MW1/1

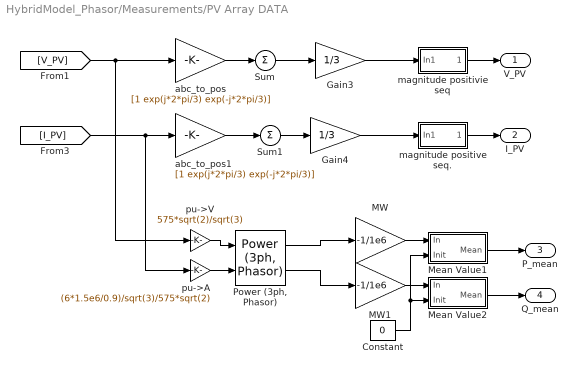
== system HybridModel_Phasor/Measurements/PV Array DATA ==
  Constant : Constant  Value=0
  Gain3 : Gain  Gain=1/3  SaturateOnIntegerOverflow=on  OutDataTypeStr=Inherit: Same as input  ParamDataTypeStr=Inherit: Same as input
  Gain4 : Gain  Gain=1/3  SaturateOnIntegerOverflow=on  OutDataTypeStr=Inherit: Same as input  ParamDataTypeStr=Inherit: Same as input
  MW : Gain  Gain=-1/1e6  SaturateOnIntegerOverflow=on  OutDataTypeStr=Inherit: Same as input  ParamDataTypeStr=Inherit: Same as input
  MW1 : Gain  Gain=-1/1e6  SaturateOnIntegerOverflow=on  OutDataTypeStr=Inherit: Same as input  ParamDataTypeStr=Inherit: Same as input
  Mean Value1 : Subsystem  mask(Mean value){Period=1/60}
      mask prompts: Period "Averaging period (s):"
      mask help: This block uses the running window averaging technique to compute the mean value of the input signal over the specified period.
  Mean Value2 : Subsystem  mask(Mean value){Period=1/60}
      mask prompts: Period "Averaging period (s):"
      mask help: This block uses the running window averaging technique to compute the mean value of the input signal over the specified period.
  "Power (3ph, Phasor)" : powerlib_meascontrol/Measurements/Power (3ph, Phasor)
      settings: SourceProductName=Simscape Electrical  SourceProductBaseCode=PS
  Sum : Sum  Inputs=1  SaturateOnIntegerOverflow=on  InputSameDT=on  OutDataTypeStr=Inherit: Same as first input
  Sum1 : Sum  Inputs=1  SaturateOnIntegerOverflow=on  InputSameDT=on  OutDataTypeStr=Inherit: Same as first input
  abc_to_pos : Gain  Gain=[1 exp(j*2*pi/3) exp(-j*2*pi/3)]  SaturateOnIntegerOverflow=on  OutDataTypeStr=Inherit: Same as input  ParamDataTypeStr=Inherit: Same as input
  abc_to_pos1 : Gain  Gain=[1 exp(j*2*pi/3) exp(-j*2*pi/3)]  SaturateOnIntegerOverflow=on  OutDataTypeStr=Inherit: Same as input  ParamDataTypeStr=Inherit: Same as input
  "magnitude positive seq. " : Subsystem
  magnitude positivie seq : Subsystem
  pu->A : Gain  Gain=(6*1.5e6/0.9)/sqrt(3)/575*sqrt(2)  SaturateOnIntegerOverflow=on  OutDataTypeStr=Inherit: Same as input  ParamDataTypeStr=Inherit: Same as input
  pu->V : Gain  Gain=575*sqrt(2)/sqrt(3)  SaturateOnIntegerOverflow=on  OutDataTypeStr=Inherit: Same as input  ParamDataTypeStr=Inherit: Same as input
  V_PV : Outport
  I_PV : Outport  Port=2
  P_mean : Outport  Port=3
  Q_mean : Outport  Port=4
  wires:
  [I_PV] -> pu->A/1, abc_to_pos1/1
  [V_PV] -> pu->V/1, abc_to_pos/1
  pu->A/1 -> "Power (3ph, Phasor)"/2
  pu->V/1 -> "Power (3ph, Phasor)"/1
  MW/1 -> Mean Value1/1(In)
  MW1/1 -> Mean Value2/1(In)
  "magnitude positive seq. "/1(Out1) -> I_PV/1
  magnitude positivie seq/1(Out1) -> V_PV/1
  abc_to_pos/1 -> Sum/1
  Sum/1 -> Gain3/1
  Sum1/1 -> Gain4/1
  Gain3/1 -> magnitude positivie seq/1(In1)
  abc_to_pos1/1 -> Sum1/1
  Gain4/1 -> "magnitude positive seq. "/1(In1)
  Mean Value1/1(Mean) -> P_mean/1
  Mean Value2/1(Mean) -> Q_mean/1
  Constant/1 -> Mean Value1/2(Init), Mean Value2/2(Init)
  "Power (3ph, Phasor)"/1 -> MW/1
  "Power (3ph, Phasor)"/2 -> MW1/1

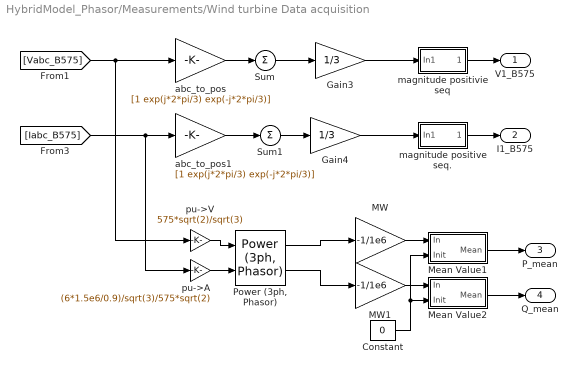
== system HybridModel_Phasor/Measurements/Wind turbine Data acquisition ==
  Constant : Constant  Value=0
  Gain3 : Gain  Gain=1/3  SaturateOnIntegerOverflow=on  OutDataTypeStr=Inherit: Same as input  ParamDataTypeStr=Inherit: Same as input
  Gain4 : Gain  Gain=1/3  SaturateOnIntegerOverflow=on  OutDataTypeStr=Inherit: Same as input  ParamDataTypeStr=Inherit: Same as input
  MW : Gain  Gain=-1/1e6  SaturateOnIntegerOverflow=on  OutDataTypeStr=Inherit: Same as input  ParamDataTypeStr=Inherit: Same as input
  MW1 : Gain  Gain=-1/1e6  SaturateOnIntegerOverflow=on  OutDataTypeStr=Inherit: Same as input  ParamDataTypeStr=Inherit: Same as input
  Mean Value1 : Subsystem  mask(Mean value){Period=1/60}
      mask prompts: Period "Averaging period (s):"
      mask help: This block uses the running window averaging technique to compute the mean value of the input signal over the specified period.
  Mean Value2 : Subsystem  mask(Mean value){Period=1/60}
      mask prompts: Period "Averaging period (s):"
      mask help: This block uses the running window averaging technique to compute the mean value of the input signal over the specified period.
  "Power (3ph, Phasor)" : powerlib_meascontrol/Measurements/Power (3ph, Phasor)
      settings: SourceProductName=Simscape Electrical  SourceProductBaseCode=PS
  Sum : Sum  Inputs=1  SaturateOnIntegerOverflow=on  InputSameDT=on  OutDataTypeStr=Inherit: Same as first input
  Sum1 : Sum  Inputs=1  SaturateOnIntegerOverflow=on  InputSameDT=on  OutDataTypeStr=Inherit: Same as first input
  abc_to_pos : Gain  Gain=[1 exp(j*2*pi/3) exp(-j*2*pi/3)]  SaturateOnIntegerOverflow=on  OutDataTypeStr=Inherit: Same as input  ParamDataTypeStr=Inherit: Same as input
  abc_to_pos1 : Gain  Gain=[1 exp(j*2*pi/3) exp(-j*2*pi/3)]  SaturateOnIntegerOverflow=on  OutDataTypeStr=Inherit: Same as input  ParamDataTypeStr=Inherit: Same as input
  "magnitude positive seq. " : Subsystem
  magnitude positivie seq : Subsystem
  pu->A : Gain  Gain=(6*1.5e6/0.9)/sqrt(3)/575*sqrt(2)  SaturateOnIntegerOverflow=on  OutDataTypeStr=Inherit: Same as input  ParamDataTypeStr=Inherit: Same as input
  pu->V : Gain  Gain=575*sqrt(2)/sqrt(3)  SaturateOnIntegerOverflow=on  OutDataTypeStr=Inherit: Same as input  ParamDataTypeStr=Inherit: Same as input
  V1_B575 : Outport
  I1_B575 : Outport  Port=2
  P_mean : Outport  Port=3
  Q_mean : Outport  Port=4
  wires:
  [Iabc_B575] -> pu->A/1, abc_to_pos1/1
  [Vabc_B575] -> pu->V/1, abc_to_pos/1
  pu->A/1 -> "Power (3ph, Phasor)"/2
  pu->V/1 -> "Power (3ph, Phasor)"/1
  MW/1 -> Mean Value1/1(In)
  MW1/1 -> Mean Value2/1(In)
  "magnitude positive seq. "/1(Out1) -> I1_B575/1
  magnitude positivie seq/1(Out1) -> V1_B575/1
  abc_to_pos/1 -> Sum/1
  Sum/1 -> Gain3/1
  Sum1/1 -> Gain4/1
  Gain3/1 -> magnitude positivie seq/1(In1)
  abc_to_pos1/1 -> Sum1/1
  Gain4/1 -> "magnitude positive seq. "/1(In1)
  Mean Value1/1(Mean) -> P_mean/1
  Mean Value2/1(Mean) -> Q_mean/1
  Constant/1 -> Mean Value1/2(Init), Mean Value2/2(Init)
  "Power (3ph, Phasor)"/1 -> MW/1
  "Power (3ph, Phasor)"/2 -> MW1/1

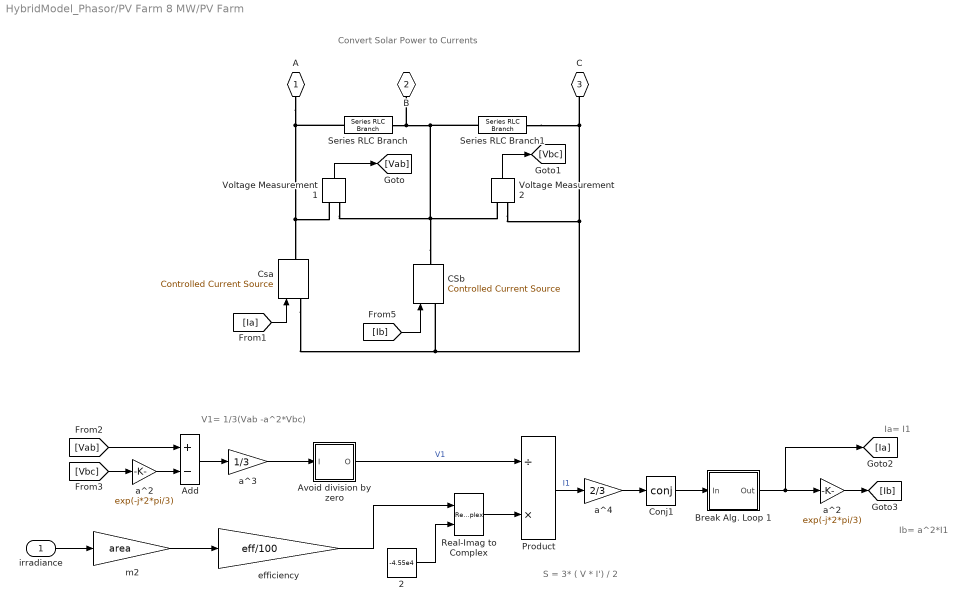
== system HybridModel_Phasor/PV Farm 8 MW/PV Farm ==
  note: Ib= a^2*I1
  note: Ia= I1
  note: S = 3* ( V * I') / 2
  note: V1= 1/3(Vab -a^2*Vbc)
  note: Convert Solar Power to Currents
  irradiance : Inport
  2 : Constant  Value=-4.55e4
  Add : Sum  Inputs=+-
  Avoid division by zero : Subsystem
  Break Alg. Loop 1 : Subsystem
  CSb : powerlib/Electrical Sources/Controlled Current Source  Initialize=on  Source_Type=AC  Amplitude=0  Phase=0  Frequency=60  Measurements=None
  Conj1 : Math  Operator=conj  SaturateOnIntegerOverflow=on
  Csa : powerlib/Electrical Sources/Controlled Current Source  Initialize=on  Source_Type=AC  Amplitude=0  Phase=0  Frequency=60  Measurements=None
  Product : Product  Inputs=/*  SaturateOnIntegerOverflow=on  InputSameDT=on  OutDataTypeStr=Inherit: Same as first input
  Real-Imag to Complex : RealImagToComplex
  Series RLC Branch : powerlib/Elements/Series RLC Branch  LConnTagsString=__new0  RConnTagsString=__new0  BranchType=R  Resistance=1e6  Inductance=1e-3  SetiL0=off  InitialCurrent=0  Capacitance=1e-6  Setx0=off  InitialVoltage=0  Measurements=None
  Series RLC Branch1 : powerlib/Elements/Series RLC Branch  LConnTagsString=__new0  RConnTagsString=__new0  BranchType=R  Resistance=1e6  Inductance=1e-3  SetiL0=off  InitialCurrent=0  Capacitance=1e-6  Setx0=off  InitialVoltage=0  Measurements=None
  Voltage Measurement1 : powerlib/Measurements/Voltage Measurement  PhasorSimulation=on  OutputType=Complex  PSBequivalent=0
  Voltage Measurement2 : powerlib/Measurements/Voltage Measurement  PhasorSimulation=on  OutputType=Complex  PSBequivalent=0
  a^2 : Gain  Gain=exp(-j*2*pi/3)  SaturateOnIntegerOverflow=on  OutDataTypeStr=Inherit: Same as input  ParamDataTypeStr=Inherit: Same as input
  "a^2 " : Gain  Gain=exp(-j*2*pi/3)  SaturateOnIntegerOverflow=on  OutDataTypeStr=Inherit: Same as input  ParamDataTypeStr=Inherit: Same as input
  a^3 : Gain  Gain=1/3  SaturateOnIntegerOverflow=on  OutDataTypeStr=Inherit: Same as input  ParamDataTypeStr=Inherit: Same as input
  a^4 : Gain  Gain=2/3  SaturateOnIntegerOverflow=on  OutDataTypeStr=Inherit: Same as input  ParamDataTypeStr=Inherit: Same as input
  efficiency : Gain  Gain=eff/100
  m2 : Gain  Gain=area
  A : PMIOPort  Tag=PMCPort  Side=Right
  B : PMIOPort  Tag=PMCPort  Port=2  Side=Right
  C : PMIOPort  Tag=PMCPort  Port=3  Side=Right
  wires:
  [Ib] -> CSb/1
  Break Alg. Loop 1/1(Out) -> a^2/1, [Ia]
  a^4/1 -> Conj1/1
  "a^2 "/1 -> Add/2
  [Vbc] -> "a^2 "/1
  [Vab] -> Add/1
  Add/1 -> a^3/1
  a^3/1 -> Avoid division by zero/1(I)
  Conj1/1 -> Break Alg. Loop 1/1(In)
  Avoid division by zero/1(O) -> Product/1  "V1"
  a^2/1 -> [Ib]
  [Ia] -> Csa/1
  Product/1 -> a^4/1  "I1"
  Real-Imag to Complex/1 -> Product/2
  Voltage Measurement2/1 -> [Vbc]
  Voltage Measurement1/1 -> [Vab]
  efficiency/1 -> Real-Imag to Complex/1
  2/1 -> Real-Imag to Complex/2
  m2/1 -> efficiency/1
  irradiance/1 -> m2/1
  connections:
  CSb/RConn1 -- Voltage Measurement1/LConn2 -- Voltage Measurement2/LConn1 -- Series RLC Branch/RConn1 -- B/RConn1 -- Series RLC Branch1/LConn1
  Voltage Measurement2/LConn2 -- Csa/LConn1 -- CSb/LConn1 -- C/RConn1 -- Series RLC Branch1/RConn1
  A/RConn1 -- Series RLC Branch/LConn1 -- Voltage Measurement1/LConn1 -- Csa/RConn1

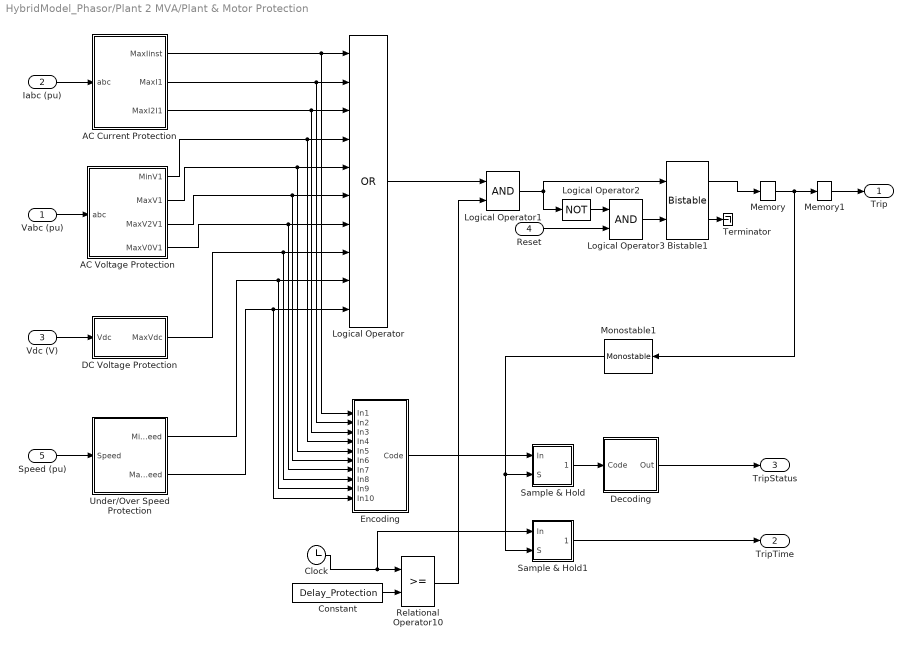
== system HybridModel_Phasor/Plant 2 MVA/Plant & Motor Protection ==
  Vabc (pu) : Inport  PortDimensions=3
  Iabc (pu) : Inport  Port=2  PortDimensions=3
  Vdc (V) : Inport  Port=3  PortDimensions=1
  Reset : Inport  Port=4  PortDimensions=1
  Speed (pu) : Inport  Port=5  PortDimensions=1
  AC Current Protection : Subsystem
  AC Voltage Protection : Subsystem
  Bistable1 : powerlib_meascontrol/Logic/Bistable  Qpriority=Set  ic=0  Ts=0
      settings: SourceProductName=Simscape Electrical  SourceProductBaseCode=PS
  Clock : Clock
  Constant : Constant  Value=Delay_Protection
  DC Voltage Protection : Subsystem
  Decoding : Subsystem
  Encoding : Subsystem
  Logical Operator : Logic  Operator=OR  Inputs=10  AllPortsSameDT=off
  Logical Operator1 : Logic  AllPortsSameDT=off
  Logical Operator2 : Logic  Operator=NOT  AllPortsSameDT=off
  Logical Operator3 : Logic  AllPortsSameDT=off
  Memory : Memory  InheritSampleTime=on
  Memory1 : Memory  InheritSampleTime=on
  Monostable1 : powerlib_meascontrol/Logic/Monostable  EdgeDetect=Rising  PulseDuration=1e-9  ic=0  Ts=0
      settings: SourceProductName=Simscape Electrical  SourceProductBaseCode=PS
  Relational Operator10 : RelationalOperator  RndMeth=Nearest
  Sample & Hold : Subsystem  DialogController=POWERSYS.PowerSysDialog  mask(Sample & Hold){ic=0}
      mask prompts: ic "Initial condition:"
      mask help: The output follows input 1 (In) as long as input 2 (S) is TRUE (1) . The output is held when input 2 becomes FALSE (0). The output initial value is specified by the parameter "Initial condition".
      mask init:
      | power_initmask();
      mask Help: This block is part of a subset of blocks in the Extras library that does not have documentation associated with it, other than the block mask description.
      mask Display: disp('S/H')
  Sample & Hold1 : Subsystem  DialogController=POWERSYS.PowerSysDialog  mask(Sample & Hold){ic=0}
      mask prompts: ic "Initial condition:"
      mask help: The output follows input 1 (In) as long as input 2 (S) is TRUE (1) . The output is held when input 2 becomes FALSE (0). The output initial value is specified by the parameter "Initial condition".
      mask init:
      | power_initmask();
      mask Help: This block is part of a subset of blocks in the Extras library that does not have documentation associated with it, other than the block mask description.
      mask Display: disp('S/H')
  Terminator : Terminator
  Under/Over Speed Protection : Subsystem
  Trip : Outport
  TripTime : Outport  Port=2
  TripStatus : Outport  Port=3
  wires:
  Memory1/1 -> Trip/1
  Vdc (V)/1 -> DC Voltage Protection/1(Vdc)
  DC Voltage Protection/1(MaxVdc) -> Logical Operator/8, Encoding/8(In8)
  Logical Operator2/1 -> Logical Operator3/1
  Reset/1 -> Logical Operator3/2
  Logical Operator3/1 -> Bistable1/2
  Logical Operator1/1 -> Bistable1/1, Logical Operator2/1
  Encoding/1(Code) -> Sample & Hold/1(In)
  Bistable1/1 -> Memory/1
  Memory/1 -> Monostable1/1, Memory1/1
  Bistable1/2 -> Terminator/1
  Sample & Hold/1("   ") -> Decoding/1(Code)
  Decoding/1(Out) -> TripStatus/1
  Iabc (pu)/1 -> AC Current Protection/1(abc)
  Vabc (pu)/1 -> AC Voltage Protection/1(abc)
  AC Current Protection/1(MaxIinst) -> Logical Operator/1, Encoding/1(In1)
  AC Current Protection/2(MaxI1) -> Logical Operator/2, Encoding/2(In2)
  AC Current Protection/3(MaxI2I1) -> Logical Operator/3, Encoding/3(In3)
  AC Voltage Protection/1(MinV1) -> Logical Operator/4, Encoding/4(In4)
  AC Voltage Protection/2(MaxV1) -> Logical Operator/5, Encoding/5(In5)
  AC Voltage Protection/3(MaxV2V1) -> Logical Operator/6, Encoding/6(In6)
  AC Voltage Protection/4(MaxV0V1) -> Logical Operator/7, Encoding/7(In7)
  Sample & Hold1/1("   ") -> TripTime/1
  Monostable1/1 -> Sample & Hold/2(S), Sample & Hold1/2(S)
  Constant/1 -> Relational Operator10/2
  Clock/1 -> Relational Operator10/1, Sample & Hold1/1(In)
  Logical Operator/1 -> Logical Operator1/1
  Relational Operator10/1 -> Logical Operator1/2
  Under/Over Speed Protection/1(MinSpeed) -> Logical Operator/9, Encoding/9(In9)
  Under/Over Speed Protection/2(MaxSpeed) -> Logical Operator/10, Encoding/10(In10)
  Speed (pu)/1 -> Under/Over Speed Protection/1(Speed)

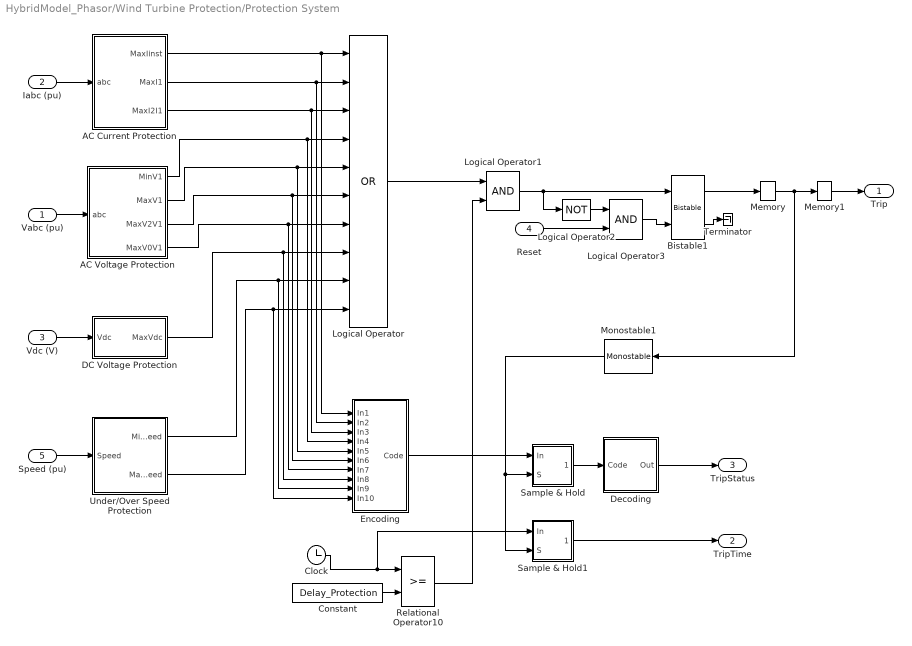
== system HybridModel_Phasor/Wind Turbine Protection/Protection System ==
  Vabc (pu) : Inport  PortDimensions=3
  Iabc (pu) : Inport  Port=2  PortDimensions=3
  Vdc (V) : Inport  Port=3  PortDimensions=1
  Reset : Inport  Port=4  PortDimensions=1
  Speed (pu) : Inport  Port=5  PortDimensions=1
  AC Current Protection : Subsystem
  AC Voltage Protection : Subsystem
  Bistable1 : powerlib_meascontrol/Logic/Bistable  Qpriority=Set  ic=0  Ts=0
      settings: SourceProductName=Simscape Electrical  SourceProductBaseCode=PS
  Clock : Clock
  Constant : Constant  Value=Delay_Protection
  DC Voltage Protection : Subsystem
  Decoding : Subsystem
  Encoding : Subsystem
  Logical Operator : Logic  Operator=OR  Inputs=10  AllPortsSameDT=off
  Logical Operator1 : Logic  AllPortsSameDT=off
  Logical Operator2 : Logic  Operator=NOT  AllPortsSameDT=off
  Logical Operator3 : Logic  AllPortsSameDT=off
  Memory : Memory  InheritSampleTime=on
  Memory1 : Memory  InheritSampleTime=on
  Monostable1 : powerlib_meascontrol/Logic/Monostable  EdgeDetect=Rising  PulseDuration=1e-9  ic=0  Ts=0
      settings: SourceProductName=Simscape Electrical  SourceProductBaseCode=PS
  Relational Operator10 : RelationalOperator  RndMeth=Nearest
  Sample & Hold : Subsystem  DialogController=POWERSYS.PowerSysDialog  mask(Sample & Hold){ic=0}
      mask prompts: ic "Initial condition:"
      mask help: The output follows input 1 (In) as long as input 2 (S) is TRUE (1) . The output is held when input 2 becomes FALSE (0). The output initial value is specified by the parameter "Initial condition".
      mask init:
      | power_initmask();
      mask Help: This block is part of a subset of blocks in the Extras library that does not have documentation associated with it, other than the block mask description.
      mask Display: disp('S/H')
  Sample & Hold1 : Subsystem  DialogController=POWERSYS.PowerSysDialog  mask(Sample & Hold){ic=0}
      mask prompts: ic "Initial condition:"
      mask help: The output follows input 1 (In) as long as input 2 (S) is TRUE (1) . The output is held when input 2 becomes FALSE (0). The output initial value is specified by the parameter "Initial condition".
      mask init:
      | power_initmask();
      mask Help: This block is part of a subset of blocks in the Extras library that does not have documentation associated with it, other than the block mask description.
      mask Display: disp('S/H')
  Terminator : Terminator
  Under/Over Speed Protection : Subsystem
  Trip : Outport
  TripTime : Outport  Port=2
  TripStatus : Outport  Port=3
  wires:
  Speed (pu)/1 -> Under/Over Speed Protection/1(Speed)
  Under/Over Speed Protection/2(MaxSpeed) -> Encoding/10(In10), Logical Operator/10
  Under/Over Speed Protection/1(MinSpeed) -> Encoding/9(In9), Logical Operator/9
  Relational Operator10/1 -> Logical Operator1/2
  Logical Operator/1 -> Logical Operator1/1
  Clock/1 -> Sample & Hold1/1(In), Relational Operator10/1
  Constant/1 -> Relational Operator10/2
  Monostable1/1 -> Sample & Hold1/2(S), Sample & Hold/2(S)
  Sample & Hold1/1("   ") -> TripTime/1
  AC Voltage Protection/4(MaxV0V1) -> Encoding/7(In7), Logical Operator/7
  AC Voltage Protection/3(MaxV2V1) -> Encoding/6(In6), Logical Operator/6
  AC Voltage Protection/2(MaxV1) -> Encoding/5(In5), Logical Operator/5
  AC Voltage Protection/1(MinV1) -> Encoding/4(In4), Logical Operator/4
  AC Current Protection/3(MaxI2I1) -> Encoding/3(In3), Logical Operator/3
  AC Current Protection/2(MaxI1) -> Encoding/2(In2), Logical Operator/2
  AC Current Protection/1(MaxIinst) -> Encoding/1(In1), Logical Operator/1
  Vabc (pu)/1 -> AC Voltage Protection/1(abc)
  Iabc (pu)/1 -> AC Current Protection/1(abc)
  Decoding/1(Out) -> TripStatus/1
  Sample & Hold/1("   ") -> Decoding/1(Code)
  Bistable1/2 -> Terminator/1
  Memory/1 -> Monostable1/1, Memory1/1
  Bistable1/1 -> Memory/1
  Encoding/1(Code) -> Sample & Hold/1(In)
  Logical Operator1/1 -> Bistable1/1, Logical Operator2/1
  Logical Operator3/1 -> Bistable1/2
  Reset/1 -> Logical Operator3/2
  Logical Operator2/1 -> Logical Operator3/1
  DC Voltage Protection/1(MaxVdc) -> Encoding/8(In8), Logical Operator/8
  Vdc (V)/1 -> DC Voltage Protection/1(Vdc)
  Memory1/1 -> Trip/1
